simulink model "Made2OrderCode"  (R2021a)
settings: Solver=FixedStepAuto  StartTime=0.0  StopTime=inf  RelTol=1e-3  EnableMultiTasking=on
libraries: vexarmcortexlib x24, vexcommonlib x5
settings Model: ExtModeTrigDuration=25  Creator=eagle  LastModifiedBy=eagle
settings OptimizationCC: EnhancedBackFolding=on  PassReuseOutputArgsAs=Individual arguments  ZeroExternalMemoryAtStartup=off  ZeroInternalMemoryAtStartup=off  MaxStackSize=64  OptimizeBlockOrder=speed  DifferentSizesBufferReuse=on  OptimizationCustomize=off  EfficientTunableParamExpr=on
settings DebuggingCC: ParameterTunabilityLossMsg=error
settings HardwareCC: ProdBitPerPointer=32  ProdBitPerSizeT=32  ProdBitPerPtrDiffT=32  ProdLargestAtomicInteger=Long  ProdLargestAtomicFloat=Double  ProdWordSize=32  ProdHWDeviceType=ARM Compatible->ARM Cortex
settings SFSimCC: MATLABDynamicMemAlloc=off
settings RTWCC: SystemTargetFile=ert.tlc  HardwareBoard=ARM Cortex-based VEX Microcontroller  TLCOptions="-aInlineSetEventsForThisBaseRateFcn=TLC_FALSE -aSuppressMultiTaskScheduler=TLC_FALSE  -aRateBasedStepFcn=0"  TemplateMakefile=ert_default_tmf  Toolchain=GNU Tools for VEX ARM Cortex
settings CodeAppCC: ForceParamTrailComments=on  IgnoreCustomStorageClasses=off  OperatorAnnotations=on  SimulinkDataObjDesc=on  SFDataObjDesc=on  InsertBlockDesc=on
settings ERTTargetCC: ExtModeTransport=1  ExtModeMexFile=ext_serial_win32_comm

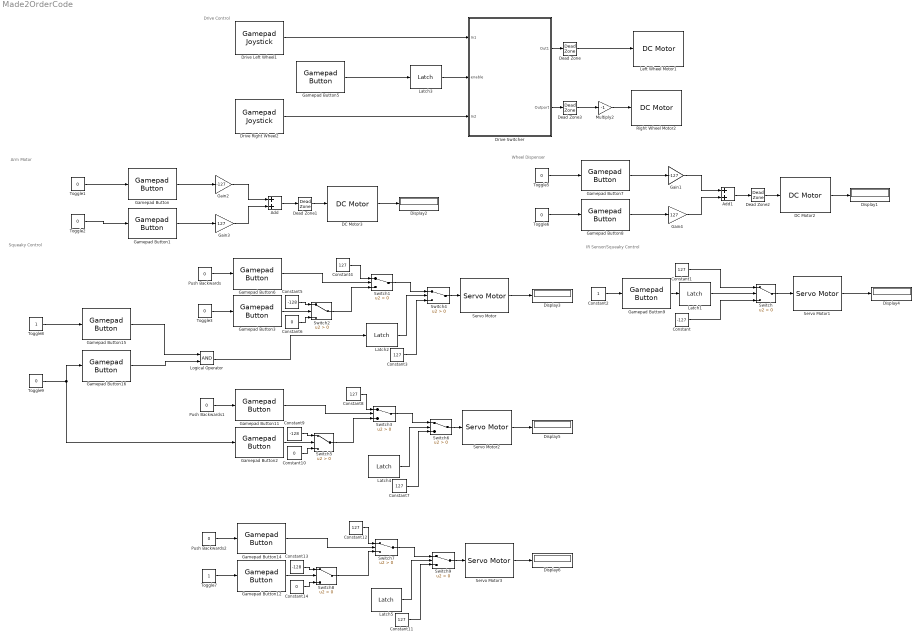
== system Made2OrderCode ==
  note: Arm Motor
  note: IR Sensor/Squeaky Control
  note: Squeaky Control
  note: Drive Control
  note: Wheel Dispenser
  Add : Sum
  Add1 : Sum
  Constant : Constant  Value=-127
  Constant{1,3..4,7..8,11..12} (7 alike) : Constant  Value=127
  Constant10 : Constant  Value=0
  Constant13 : Constant  Value=-128
  Constant14 : Constant  Value=0
  Constant2 : Constant
  Constant5 : Constant  Value=-128
  Constant6 : Constant  Value=0
  Constant9 : Constant  Value=-128
  DC Motor2 : vexarmcortexlib/Actuators/DC Motor  motor=7  scaleFactor=1/13.5  SimulationOut=on
      settings: SourceProductBaseCode=EC_VEX_MICRO
  DC Motor3 : vexarmcortexlib/Actuators/DC Motor  motor=4  scaleFactor=1/13.5  SimulationOut=on
      settings: SourceProductBaseCode=EC_VEX_MICRO
  Dead Zone{,1..3} (4 alike) : DeadZone  LowerValue=-10  UpperValue=10  SaturateOnIntegerOverflow=on
  Display{1..6} (6 alike) : Display
  Drive Left Wheel1 : vexarmcortexlib/Gamepad/Gamepad Joystick  joystick=1  chan=2  SimulationIn=off  SampleTime=0.02
      settings: SourceProductBaseCode=EC_VEX_MICRO
  Drive Right Wheel2 : vexarmcortexlib/Gamepad/Gamepad Joystick  joystick=1  chan=3  SimulationIn=off  SampleTime=0.02
      settings: SourceProductBaseCode=EC_VEX_MICRO
  Drive Switcher : Subsystem  TreatAsAtomicUnit=on
  Gain1 : Gain  Gain=-127
  Gain2 : Gain  Gain=-127
  Gain3 : Gain  Gain=127
  Gain4 : Gain  Gain=127
  Gamepad Button : vexarmcortexlib/Gamepad/Gamepad Button  joystick=1  chan=5  button56=Up  button78=Down  SimulationIn=on  SampleTime=0.02
      settings: SourceProductBaseCode=EC_VEX_MICRO
  Gamepad Button1 : vexarmcortexlib/Gamepad/Gamepad Button  joystick=1  chan=6  button56=Up  button78=Up  SimulationIn=on  SampleTime=0.02
      settings: SourceProductBaseCode=EC_VEX_MICRO
  Gamepad Button11 : vexarmcortexlib/Gamepad/Gamepad Button  joystick=1  chan=7  button56=Up  button78=Left  SimulationIn=on  SampleTime=0.02
      settings: SourceProductBaseCode=EC_VEX_MICRO
  Gamepad Button12 : vexarmcortexlib/Gamepad/Gamepad Button  joystick=1  chan=5  button56=Down  button78=Down  SimulationIn=on  SampleTime=0.02
      settings: SourceProductBaseCode=EC_VEX_MICRO
  Gamepad Button14 : vexarmcortexlib/Gamepad/Gamepad Button  joystick=1  chan=5  button56=Up  button78=Up  SimulationIn=on  SampleTime=0.02
      settings: SourceProductBaseCode=EC_VEX_MICRO
  Gamepad Button15 : vexarmcortexlib/Gamepad/Gamepad Button  joystick=1  chan=7  button56=Up  button78=Down  SimulationIn=on  SampleTime=0.02
      settings: SourceProductBaseCode=EC_VEX_MICRO
  Gamepad Button16 : vexarmcortexlib/Gamepad/Gamepad Button  joystick=1  chan=7  button56=Up  button78=Right  SimulationIn=on  SampleTime=0.02
      settings: SourceProductBaseCode=EC_VEX_MICRO
  Gamepad Button2 : vexarmcortexlib/Gamepad/Gamepad Button  joystick=1  chan=7  button56=Up  button78=Right  SimulationIn=on  SampleTime=0.02
      settings: SourceProductBaseCode=EC_VEX_MICRO
  Gamepad Button3 : vexarmcortexlib/Gamepad/Gamepad Button  joystick=1  chan=7  button56=Up  button78=Down  SimulationIn=on  SampleTime=0.02
      settings: SourceProductBaseCode=EC_VEX_MICRO
  Gamepad Button5 : vexarmcortexlib/Gamepad/Gamepad Button  joystick=1  chan=8  button56=Up  button78=Down  SimulationIn=off  SampleTime=0.02
      settings: SourceProductBaseCode=EC_VEX_MICRO
  Gamepad Button6 : vexarmcortexlib/Gamepad/Gamepad Button  joystick=1  chan=7  button56=Up  button78=Up  SimulationIn=on  SampleTime=0.02
      settings: SourceProductBaseCode=EC_VEX_MICRO
  Gamepad Button7 : vexarmcortexlib/Gamepad/Gamepad Button  joystick=1  chan=8  button56=Up  button78=Left  SimulationIn=on  SampleTime=0.02
      settings: SourceProductBaseCode=EC_VEX_MICRO
  Gamepad Button8 : vexarmcortexlib/Gamepad/Gamepad Button  joystick=1  chan=8  button56=Up  button78=Right  SimulationIn=on  SampleTime=0.02
      settings: SourceProductBaseCode=EC_VEX_MICRO
  Gamepad Button9 : vexarmcortexlib/Gamepad/Gamepad Button  joystick=1  chan=8  button56=Up  button78=Up  SimulationIn=on  SampleTime=0.02
      settings: SourceProductBaseCode=EC_VEX_MICRO
  Latch{1..5} (5 alike) : vexcommonlib/Latch  output0=off  BlockPlatform=vexarmcortex
      settings: SourceProductBaseCode=EC_VEX_MICRO,VEXV5
  Left Wheel Motor1 : vexarmcortexlib/Actuators/DC Motor  motor=2  scaleFactor=1/13.5  SimulationOut=off
      settings: SourceProductBaseCode=EC_VEX_MICRO
  Logical Operator : Logic  AllPortsSameDT=off  OutDataTypeStr=boolean
  Multiply2 : Gain  Gain=-1
  Push Backwards : Constant  Value=0
      settings: OpenFcn=|
      | if strcmp('0',get_param(gcb, 'Value'))                        set_param(gcb, 'Value', '1');
      | else
      |             set_param(gcb, 'Value', '0');
      | end
  Push Backwards1 : Constant  Value=0
      settings: OpenFcn=|
      | if strcmp('0',get_param(gcb, 'Value'))                        set_param(gcb, 'Value', '1');
      | else
      |             set_param(gcb, 'Value', '0');
      | end
  Push Backwards2 : Constant  Value=0
      settings: OpenFcn=|
      | if strcmp('0',get_param(gcb, 'Value'))                        set_param(gcb, 'Value', '1');
      | else
      |             set_param(gcb, 'Value', '0');
      | end
  Right Wheel Motor2 : vexarmcortexlib/Actuators/DC Motor  motor=3  scaleFactor=1/13.5  SimulationOut=off
      settings: SourceProductBaseCode=EC_VEX_MICRO
  Servo Motor : vexarmcortexlib/Actuators/Servo Motor  motor=9  scaleFactor=60/127  SimulationOut=on
      settings: SourceProductBaseCode=EC_VEX_MICRO
  Servo Motor1 : vexarmcortexlib/Actuators/Servo Motor  motor=5  scaleFactor=60/127  SimulationOut=on
      settings: SourceProductBaseCode=EC_VEX_MICRO
  Servo Motor2 : vexarmcortexlib/Actuators/Servo Motor  motor=8  scaleFactor=60/127  SimulationOut=on
      settings: SourceProductBaseCode=EC_VEX_MICRO
  Servo Motor3 : vexarmcortexlib/Actuators/Servo Motor  motor=10  scaleFactor=60/127  SimulationOut=on
      settings: SourceProductBaseCode=EC_VEX_MICRO
  Switch{,1..9} (10 alike) : Switch  Criteria=u2 > Threshold
  Toggle{1..3,5..6,9} (6 alike) : Constant  Value=0
      settings: OpenFcn=|
      | if strcmp('0',get_param(gcb, 'Value'))                        set_param(gcb, 'Value', '1');
      | else
      |             set_param(gcb, 'Value', '0');
      | end
  Toggle7 : Constant
      settings: OpenFcn=|
      | if strcmp('0',get_param(gcb, 'Value'))                        set_param(gcb, 'Value', '1');
      | else
      |             set_param(gcb, 'Value', '0');
      | end
  Toggle8 : Constant
      settings: OpenFcn=|
      | if strcmp('0',get_param(gcb, 'Value'))                        set_param(gcb, 'Value', '1');
      | else
      |             set_param(gcb, 'Value', '0');
      | end
  wires:
  Gain3/1 -> Add/2
  Gain2/1 -> Add/1
  DC Motor3/1 -> Display2/1
  Push Backwards/1 -> Gamepad Button6/1
  Toggle2/1 -> Gamepad Button1/1
  Toggle1/1 -> Gamepad Button/1
  Gamepad Button9/1 -> Latch1/1
  Servo Motor1/1 -> Display4/1
  Toggle3/1 -> Gamepad Button3/1
  Constant2/1 -> Gamepad Button9/1
  Constant/1 -> Switch/3
  Constant1/1 -> Switch/1
  Drive Switcher/2(Outport) -> Dead Zone3/1
  Drive Switcher/1(Out1) -> Dead Zone/1
  Drive Right Wheel2/1 -> Drive Switcher/3(In2)
  Latch3/1 -> Drive Switcher/2(enable)
  Drive Left Wheel1/1 -> Drive Switcher/1(In1)
  Gamepad Button5/1 -> Latch3/1
  Add/1 -> Dead Zone1/1
  Gamepad Button1/1 -> Gain3/1
  Gamepad Button/1 -> Gain2/1
  Dead Zone1/1 -> DC Motor3/1
  Switch1/1 -> Switch4/1
  Gamepad Button3/1 -> Switch2/2
  Constant5/1 -> Switch2/1
  Constant6/1 -> Switch2/3
  Servo Motor/1 -> Display3/1
  Gamepad Button6/1 -> Switch1/2
  Gamepad Button8/1 -> Gain4/1
  Gamepad Button7/1 -> Gain1/1
  Dead Zone2/1 -> DC Motor2/1
  DC Motor2/1 -> Display1/1
  Add1/1 -> Dead Zone2/1
  Gain1/1 -> Add1/1
  Toggle6/1 -> Gamepad Button8/1
  Toggle5/1 -> Gamepad Button7/1
  Gain4/1 -> Add1/2
  Switch/1 -> Servo Motor1/1
  Constant4/1 -> Switch1/1
  Switch2/1 -> Switch1/3
  Latch1/1 -> Switch/2
  Latch2/1 -> Switch4/2
  Constant3/1 -> Switch4/3
  Switch4/1 -> Servo Motor/1
  Constant8/1 -> Switch3/1
  Switch6/1 -> Servo Motor2/1
  Constant7/1 -> Switch6/3
  Latch4/1 -> Switch6/2
  Switch5/1 -> Switch3/3
  Switch3/1 -> Switch6/1
  Toggle9/1 -> Gamepad Button2/1, Gamepad Button16/1
  Constant10/1 -> Switch5/3
  Constant9/1 -> Switch5/1
  Gamepad Button2/1 -> Switch5/2
  Push Backwards1/1 -> Gamepad Button11/1
  Gamepad Button11/1 -> Switch3/2
  Constant12/1 -> Switch7/1
  Switch9/1 -> Servo Motor3/1
  Constant11/1 -> Switch9/3
  Latch5/1 -> Switch9/2
  Switch8/1 -> Switch7/3
  Switch7/1 -> Switch9/1
  Toggle7/1 -> Gamepad Button12/1
  Constant14/1 -> Switch8/3
  Logical Operator/1 -> Latch2/1
  Constant13/1 -> Switch8/1
  Gamepad Button12/1 -> Switch8/2
  Push Backwards2/1 -> Gamepad Button14/1
  Gamepad Button14/1 -> Switch7/2
  Servo Motor2/1 -> Display5/1
  Servo Motor3/1 -> Display6/1
  Gamepad Button15/1 -> Logical Operator/1
  Gamepad Button16/1 -> Logical Operator/2
  Toggle8/1 -> Gamepad Button15/1
  Dead Zone3/1 -> Multiply2/1
  Multiply2/1 -> Right Wheel Motor2/1
  Dead Zone/1 -> Left Wheel Motor1/1

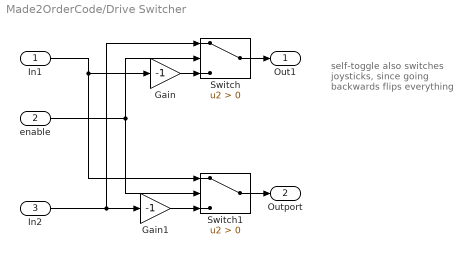
== system Made2OrderCode/Drive Switcher ==
  note: self-toggle also switches joysticks, since going backwards flips everything
  In1 : Inport
  enable : Inport  Port=2
  In2 : Inport  Port=3
  Gain : Gain  Gain=-1
  Gain1 : Gain  Gain=-1
  Switch : Switch  Criteria=u2 > Threshold
  Switch1 : Switch  Criteria=u2 > Threshold
  Out1 : Outport
  Outport : Outport  Port=2
  wires:
  Switch/1 -> Out1/1
  Switch1/1 -> Outport/1
  enable/1 -> Switch/2, Switch1/2
  In1/1 -> Gain/1, Switch1/1
  In2/1 -> Gain1/1, Switch/1
  Gain/1 -> Switch/3
  Gain1/1 -> Switch1/3
